simulink model "Code_Gen_Model"  (R2023a)
settings: Solver=FixedStepDiscrete  StartTime=0.0  StopTime=inf  FixedStep=t_sample  RelTol=1e-3
libraries: Code_Gen_lib x1
settings Model: Creator=FIRSTMentor  LastModifiedBy=FIRSTMentor
settings OptimizationCC: DefaultParameterBehavior=Inlined  StrengthReduction=on  PassReuseOutputArgsAs=Individual arguments  ZeroExternalMemoryAtStartup=off  ZeroInternalMemoryAtStartup=off  OptimizeBlockOrder=speed  OptimizationPriority=Speed  OptimizationCustomize=off  MultiThreadedLoops=on  EfficientTunableParamExpr=on
settings DebuggingCC: UnderspecifiedInitializationDetection=Classic  MergeDetectMultiDrivingBlocksExec=none  ParameterTunabilityLossMsg=error
settings ModelReferenceCC: PropagateSignalLabelsOutOfModel=off
settings SFSimCC: MATLABDynamicMemAlloc=off
settings RTWCC: Description=Embedded Coder  SystemTargetFile=ert.tlc  GenCodeOnly=on  TemplateMakefile=ert_default_tmf  Toolchain=Microsoft Visual C++ 2022 v17.0 | CMake/nmake (64-bit Windows)  BuildConfiguration=Release
settings CodeAppCC: ForceParamTrailComments=on  IgnoreCustomStorageClasses=off  OperatorAnnotations=on  SimulinkDataObjDesc=on  SFDataObjDesc=on  InsertBlockDesc=on
settings ERTTargetCC: TargetLangStandard=C99 (ISO)  GenerateSampleERTMain=on  ParenthesesLevel=Minimum  InlinedParameterPlacement=NonHierarchical  ERTCustomFileTemplate=example_file_process.tlc

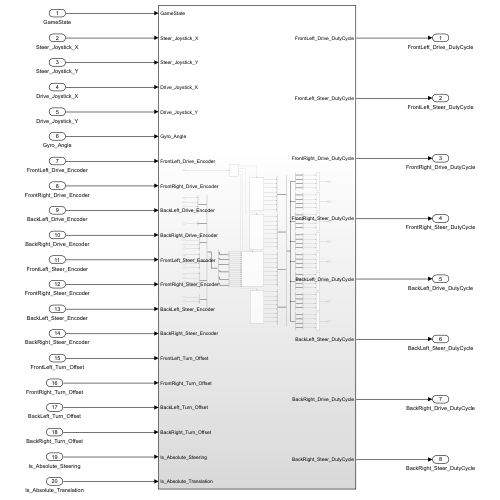
[thumbnail: Simulink's stored preview of the top-level diagram]
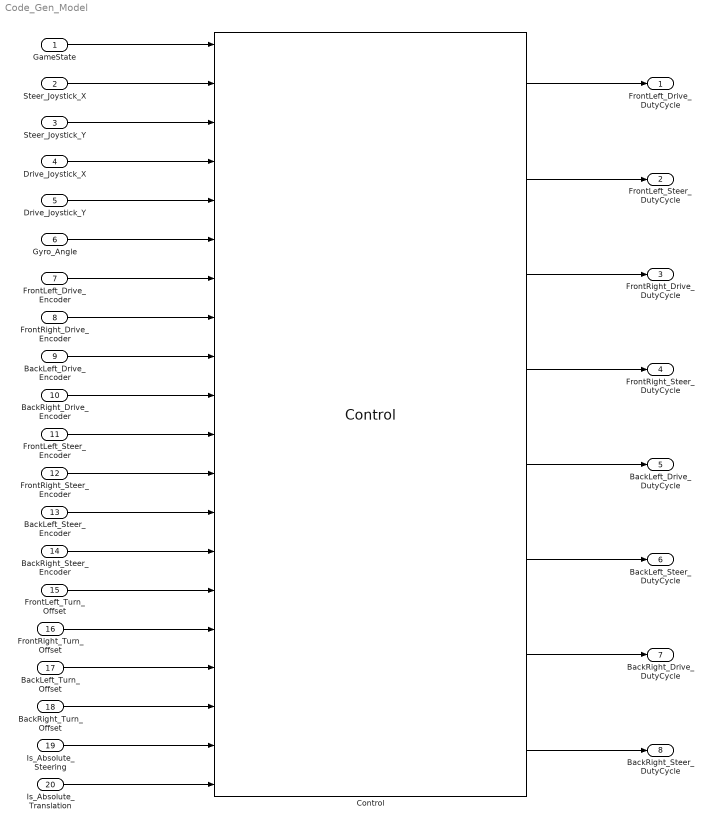
== system Code_Gen_Model ==
  GameState : Inport
  Steer_Joystick_X : Inport  Port=2
  Steer_Joystick_Y : Inport  Port=3
  Drive_Joystick_X : Inport  Port=4
  Drive_Joystick_Y : Inport  Port=5
  Gyro_Angle : Inport  Port=6
  FrontLeft_Drive_Encoder : Inport  Port=7
  FrontRight_Drive_Encoder : Inport  Port=8
  BackLeft_Drive_Encoder : Inport  Port=9
  BackRight_Drive_Encoder : Inport  Port=10
  FrontLeft_Steer_Encoder : Inport  Port=11
  FrontRight_Steer_Encoder : Inport  Port=12
  BackLeft_Steer_Encoder : Inport  Port=13
  BackRight_Steer_Encoder : Inport  Port=14
  FrontLeft_Turn_Offset : Inport  Port=15
  FrontRight_Turn_Offset : Inport  Port=16
  BackLeft_Turn_Offset : Inport  Port=17
  BackRight_Turn_Offset : Inport  Port=18
  Is_Absolute_Steering : Inport  Port=19
  Is_Absolute_Translation : Inport  Port=20
  Control : Code_Gen_lib/Control  SystemSampleTime=-1  VariantActivationTime=update diagram  Latency=0  AutoFrameSizeCalculation=off
  FrontLeft_Drive_DutyCycle : Outport
  FrontLeft_Steer_DutyCycle : Outport  Port=2
  FrontRight_Drive_DutyCycle : Outport  Port=3
  FrontRight_Steer_DutyCycle : Outport  Port=4
  BackLeft_Drive_DutyCycle : Outport  Port=5
  BackLeft_Steer_DutyCycle : Outport  Port=6
  BackRight_Drive_DutyCycle : Outport  Port=7
  BackRight_Steer_DutyCycle : Outport  Port=8
  wires:
  GameState/1 -> Control/1
  Steer_Joystick_X/1 -> Control/2
  Steer_Joystick_Y/1 -> Control/3
  Drive_Joystick_X/1 -> Control/4
  Drive_Joystick_Y/1 -> Control/5
  Gyro_Angle/1 -> Control/6
  FrontLeft_Drive_Encoder/1 -> Control/7
  FrontRight_Drive_Encoder/1 -> Control/8
  BackLeft_Drive_Encoder/1 -> Control/9
  BackRight_Drive_Encoder/1 -> Control/10
  FrontLeft_Steer_Encoder/1 -> Control/11
  FrontRight_Steer_Encoder/1 -> Control/12
  BackLeft_Steer_Encoder/1 -> Control/13
  BackRight_Steer_Encoder/1 -> Control/14
  Control/1 -> FrontLeft_Drive_DutyCycle/1
  Control/2 -> FrontLeft_Steer_DutyCycle/1
  Control/3 -> FrontRight_Drive_DutyCycle/1
  Control/4 -> FrontRight_Steer_DutyCycle/1
  Control/5 -> BackLeft_Drive_DutyCycle/1
  Control/6 -> BackLeft_Steer_DutyCycle/1
  Control/7 -> BackRight_Drive_DutyCycle/1
  Control/8 -> BackRight_Steer_DutyCycle/1
  FrontLeft_Turn_Offset/1 -> Control/15
  FrontRight_Turn_Offset/1 -> Control/16
  BackLeft_Turn_Offset/1 -> Control/17
  BackRight_Turn_Offset/1 -> Control/18
  Is_Absolute_Steering/1 -> Control/19
  Is_Absolute_Translation/1 -> Control/20
